simulink model "W04_LowPass"  (R2024b)
settings: Solver=ode45  StartTime=0.0  StopTime=t_end  MaxStep=0.01  RelTol=1e-3
PreLoadFcn:
  | % W04_LowPass 기본 파라미터 (모델을 열 때 자동 실행)
  | defs = { 'tau',1 ; 'w_lo',0.2 ; 'w_hi',10 ; 'a_lo',1 ; 'a_hi',0.5 ; 't_end',60 };
  | for ii = 1:size(defs,1)
  |     if ~evalin('base', sprintf('exist(''%s'',''var'')', defs{ii,1}))
  |         assignin('base', defs{ii,1}, defs{ii,2});
  |     end
  | end
  | clear defs ii
values from neighbouring files (symbols this model uses):
  a_hi = 0.5    [W04_04_run_lowpass.m]
  a_lo = 1    [W04_04_run_lowpass.m]
  tau = tau_list(i)    [W04_01_first_second_order.m]    (also in W04_04_run_lowpass.m = 1)
  w_hi = 10    [W04_04_run_lowpass.m]
  w_lo = 0.2    [W04_04_run_lowpass.m]
settings Model: Creator=admin  LastModifiedBy=admin

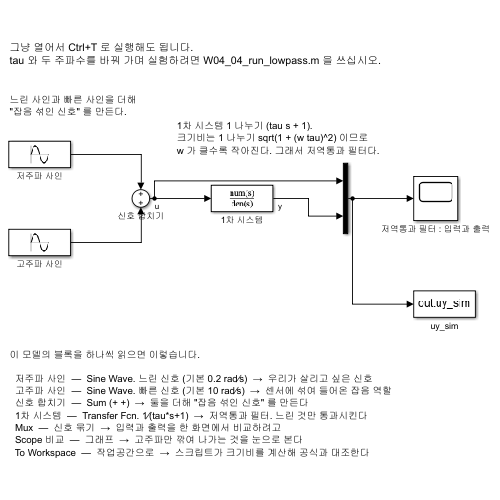
[thumbnail: Simulink's stored preview of the top-level diagram]
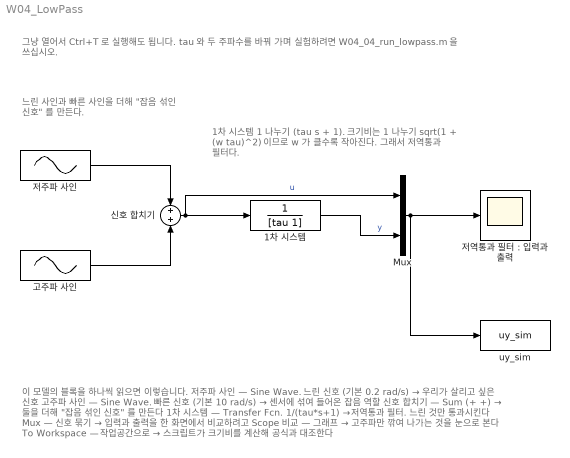
== system W04_LowPass ==
  note: 느린 사인과 빠른 사인을 더해
      | "잡음 섞인 신호" 를 만든다.
  note: 1차 시스템 1 나누기 (tau s + 1).
      | 크기비는 1 나누기 sqrt(1 + (w tau)^2) 이므로
      | w 가 클수록 작아진다. 그래서 저역통과 필터다.
  note: 그냥 열어서 Ctrl+T 로 실행해도 됩니다.
      | tau 와 두 주파수를 바꿔 가며 실험하려면 W04_04_run_lowpass.m 을 쓰십시오.
  note: 이 모델의 블록을 하나씩 읽으면 이렇습니다.
      |
      |   저주파 사인  —  Sine Wave. 느린 신호 (기본 0.2 rad∕s)  →  우리가 살리고 싶은 신호
      |   고주파 사인  —  Sine Wave. 빠른 신호 (기본 10 rad∕s)  →  센서에 섞여 들어온 잡음 역할
      |   신호 합치기  —  Sum (+ +)  →  둘을 더해 "잡음 섞인 신호" 를 만든다
      |   1차 시스템  —  Transfer Fcn. 1∕(tau*s+1)  →  저역통과 필터. 느린 것만 통과시킨다
      |   Mux  —  신호 묶기  →  입력과 출력을 한 화면에서 비교하려고
      |   Scope 비교  —  그래프  →  고주파만 깎여 나가는 것을 눈으로 본다
      |   To Workspace  —  작업공간으로  →  스크립트가 크기비를 계산해 공식과 대조한다
  1차 시스템 : TransferFcn  Denominator=[tau 1]
  Mux : Mux  Inputs=2
  uy_sim : ToWorkspace  VariableName=uy_sim  SaveFormat=Timeseries  SampleTime=-1
  고주파 사인 : Sin  Amplitude=a_hi  Frequency=w_hi  SampleTime=0
  신호 합치기 : Sum
  "저역통과 필터 : 입력과 출력" : Scope
  저주파 사인 : Sin  Amplitude=a_lo  Frequency=w_lo  SampleTime=0
  wires:
  저주파 사인/1 -> 신호 합치기/1
  고주파 사인/1 -> 신호 합치기/2
  신호 합치기/1 -> 1차 시스템/1, Mux/1  "u"
  1차 시스템/1 -> Mux/2  "y"
  Mux/1 -> "저역통과 필터 : 입력과 출력"/1, uy_sim/1
